simulink model "quantized_frequency"  (R2016a)
settings: Solver=VariableStepAuto  StartTime=0.0  StopTime=8000  RelTol=1e-3
libraries: simulink x1
settings Model: Creator=Eduardo  LastModifiedBy=Eduardo

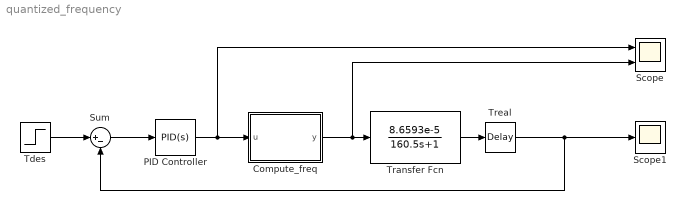
== system quantized_frequency ==
  Compute_freq : MATLAB Function  TreatAsAtomicUnit=on
  PID Controller : simulink/Continuous/PID Controller  Controller=PID  TimeDomain=Continuous-time  SampleTime=-1  IntegratorMethod=Forward Euler  FilterMethod=Forward Euler  Form=Parallel  UseFilter=on  ControllerParametersSource=internal  P=1000  I=80  D=0  N=100  InitialConditionSource=internal  InitialConditionForIntegrator=0  InitialConditionForFilter=0  ExternalReset=none  LimitOutput=off  UpperSaturationLimit=inf  LowerSaturationLimit=-inf  LinearizeAsGain=on  AntiWindupMode=none  Kb=1  TrackingMode=off  Kt=1  PParamMin=[]  PParamMax=[]  IParamMin=[]  IParamMax=[]  DParamMin=[]  DParamMax=[]  NParamMin=[]  NParamMax=[]  KbParamMin=[]  KbParamMax=[]  KtParamMin=[]  KtParamMax=[]  POutMin=[]  POutMax=[]  IOutMin=[]  IOutMax=[]  DOutMin=[]  DOutMax=[]  NOutMin=[]  NOutMax=[]  KbOutMin=[]  KbOutMax=[]  KtOutMin=[]  KtOutMax=[]  IntegratorOutMin=[]  IntegratorOutMax=[]  FilterOutMin=[]  FilterOutMax=[]  SumOutMin=[]  SumOutMax=[]  SumI1OutMin=[]  SumI1OutMax=[]  SumI2OutMin=[]  SumI2OutMax=[]  SumI3OutMin=[]  SumI3OutMax=[]  SumDOutMin=[]  SumDOutMax=[]  SaturationOutMin=[]  SaturationOutMax=[]  IntegratorContinuousStateAttributes=''  IntegratorStateMustResolveToSignalObject=off  IntegratorRTWStateStorageClass=Auto  FilterContinuousStateAttributes=''  FilterStateMustResolveToSignalObject=off  FilterRTWStateStorageClass=Auto  DifferentiatorICPrevScaledInput=0  DifferentiatorOutMin=[]  DifferentiatorOutMax=[]
  Scope : Scope  NumInputPorts=2
  Scope1 : Scope
  Sum : Sum  Inputs=|+-
  Tdes : Step  Time=0  After=75  SampleTime=0
  Transfer Fcn : TransferFcn  Numerator=[8.6593e-5]  Denominator=[160.5 1]
  Treal : TransportDelay  DelayTime=0.498
  wires:
  Compute_freq/1(y) -> Scope/2, Transfer Fcn/1
  Tdes/1 -> Sum/1
  Sum/1 -> PID Controller/1
  PID Controller/1 -> Scope/1, Compute_freq/1(u)
  Transfer Fcn/1 -> Treal/1
  Treal/1 -> Scope1/1, Sum/2

== matlab function quantized_frequency/Compute_freq ==
  data: u input; y output
function y = fcn(u)
%#codegen
freqs = [384000,
    486000,
    594000,
    702000,
    810000
    918000];
f=1;
fmax = size(freqs,1);
while (f<fmax) && (freqs(f) < u)
    f = f+1;
end
y = freqs(f);
% y = u;

% if u < 486000
%     y = 384000;
% elseif (u>=486000) && (u<550000)
%     y = 450000;
% else
%     y = 650000;
% end
